simulink model "LinkageC"  (R2025b)
settings: Solver=VariableStepAuto  StartTime=0  StopTime=numPeriods*T  RelTol=1e-3  AbsTol=1e-3
values from neighbouring files (symbols this model uses):
  A_G = 56.801    [LinkageGeometrySetUp.m]    (also in LinkageGeometrySetUp_imp.m = 55; LinkageGeometry_Fabio_ver.m = 20)
  alpha_0 = deg2rad(0.5)    [Iteration.m]    (also in Iteration_geometry.m; StartUp.m)
  alpha_stall_static = deg2rad(13)    [Iteration.m]    (also in Iteration_geometry.m; StartUp.m)
  AR = b^2/A    [LinkageGeometry_Modify.m]    (also in StartUp.m)
  Cd_cf = 1.5    [Iteration.m]    (also in Iteration_geometry.m; StartUp.m)
  CordOut = linspace(CordOut_root, CordOut_tip, WingSecNum_Out)    [LinkageGeometry_Modify.m]    (also in StartUp.m)
  D = 0;" newline      "    return;" newline      "end" newline      "q = 0.5*rho*Vmag^2;" newline      "D = q*S*CD;" newline      "L = q*S*CL;" newline      "    [build_wing_template.m]
  del_t = t_tot/(numSample)    [InputSetUp.m]
  eta_s = 0.90    (= 0.9)    [Iteration.m]    (also in Iteration_geometry.m; StartUp.m)
  InboardCord = 0.35*L_D/0.037    [LinkageGeometry_Modify.m]    (also in StartUp.m = 0.4)
  k_inboard = k * InboardCord/meanCord    [LinkageGeometry_Modify.m]    (also in StartUp.m = 12.5663706144)
  k_outboard = k * CordOut/meanCord    [LinkageGeometry_Modify.m]    (also in StartUp.m)
  Ka = 10    [StartUp3_control.m]
  Km = 73    [StartUp3_control.m]
  L_C = (3.589/1.5)*L_D    [LinkageGeometrySetUp.m]    (also in LinkageGeometrySetUp_imp.m = (9.37/3.7)*L_D; LinkageGeometry_Fabio_ver.m = 0.07885)
  L_C1 = (2.445/1.5)*L_D    [LinkageGeometrySetUp.m]    (also in LinkageGeometrySetUp_imp.m = (5.91/3.7)*L_D; LinkageGeometry_Fabio_ver.m = 0.04893)
  L_D = L_D_val(iter)    [Iteration_geometry.m]    (also in LinkageGeometry_Fabio_ver.m = 0.03019; StartUp.m = 0.037)
  L_EF = (1.494/1.5)*L_D    [LinkageGeometrySetUp.m]    (also in LinkageGeometrySetUp_imp.m = (4.468/3.7)*L_D; LinkageGeometry_Fabio_ver.m = 0.036)
  L_EG = (1.265/1.5)*L_D    [LinkageGeometrySetUp.m]    (also in LinkageGeometrySetUp_imp.m = L_C2; LinkageGeometry_Fabio_ver.m = 0.03)
  L_F = (16.189/1.5)*L_D    [LinkageGeometrySetUp.m]    (also in LinkageGeometrySetUp_imp.m = (39.93/3.7)*L_D; LinkageGeometry_Fabio_ver.m = 0.364)
  L_FH = (1.002/1.5)*L_D    [LinkageGeometrySetUp.m]    (also in LinkageGeometrySetUp_imp.m = (2.842/3.7)*L_D; LinkageGeometry_Fabio_ver.m = 0.02)
  L_Fl = (16.118/1.5)*L_D    [LinkageGeometrySetUp.m]    (also in LinkageGeometrySetUp_imp.m = L_F; LinkageGeometry_Fabio_ver.m = 0.364)
  L_Fp = (4.051/1.5)*L_D    [LinkageGeometrySetUp.m]    (also in LinkageGeometrySetUp_imp.m = (9.99/3.7)*L_D; LinkageGeometry_Fabio_ver.m = 0.14288)
  L_GH = (1.129/1.5)*L_D    [LinkageGeometrySetUp.m]    (also in LinkageGeometrySetUp_imp.m = (3.046/3.7)*L_D; LinkageGeometry_Fabio_ver.m = 0.016)
  L_t = 0.5/100    (= 0.005)    [LinkageGeometrySetUp.m]    (also in LinkageGeometrySetUp_imp.m; LinkageGeometry_Fabio_ver.m; LinkageGeometry_Modify.m)
  L_tip = (19.334/1.5)*L_D    [LinkageGeometrySetUp.m]    (also in LinkageGeometrySetUp_imp.m = (43/3.7)*L_D; LinkageGeometry_Fabio_ver.m = 0.55)
  M_in_i = M_in/WingSecNum_In    (= 0.0341666666667)    [StartUp.m]
  M_ser = 0.02    [StartUp.m]
  mu = 1.81e-5    (= 1.81e-05)    [Iteration.m]    (also in Iteration_geometry.m; StartUp.m)
  noise_freq_cutoff = 20*ang_freq    [InputSetUp.m]
  P_ref = 10    [StartUp3_control.m]
  phase_data_lookup = phase_data_lookup(1:(end-1))    [StartUp.m]
  pitch_data_lookup = pitch_ts.Data(1:numSampPerT)    [InputSetUp.m]
  pitch_gain = linspace(0.1, 1, WingSecNum_Out)    [InputSetUp.m]
  pitch_lookup_input = 1    [Iteration.m]    (also in Iteration_geometry.m; StartUp.m)
  pitch_mean = deg2rad(20)    [Iteration.m]    (also in Iteration_geometry.m; Iteration_speed.m; StartUp.m = deg2rad(1); StartUp3_control.m = deg2rad(1))
  rho = 1.225    [StartUp.m]
  SectionWidth_In = L_Inboard/WingSecNum_In    [LinkageGeometry_Modify.m]    (also in StartUp.m = (L_Inboard/WingSecNum_In)*0.6)
  SectionWidth_Out = L_outboard/WingSecNum_Out    [LinkageGeometry_Modify.m]    (also in StartUp.m)
  SpeedControlYes = 1    [StartUp3_control.m]
  TorqueLimit = 7.2    [StartUp3_control.m]
  U = 0.1    [Iteration.m]    (also in Iteration_geometry.m; StartUp.m)
  xi = 0.0    (= 0)    [Iteration.m]    (also in Iteration_geometry.m; StartUp.m)
undefined symbols (not defined in the file or in its folder): angle_data_lookup, DiscIntNeverNeededParam, magnitude, Pivot, X, Y, Z
libraries: sm_lib x1370, nesl_utility x916, simulink x478, cstblocks x78, simulink_extras x10, slpidlib x2
(part 41 of 57)

== system LinkageC/Wing System (Festo)/Wing Tip/WingSeg_Out_6/1993dL&dT ==
  i : Inport
  inboard_yes? : Inport  Port=2
  AeroCalc : MATLAB Function  TreatAsAtomicUnit=on
  Discrete Derivative : simulink/Discrete/Discrete Derivative  gainval=1.0  ICPrevScaledInput=0.0  OutMin=[]  OutMax=[]  OutDataType=fixdt(1, 16)  OutScaling=2^-10  DoSatur=off
  Discrete Derivative1 : simulink/Discrete/Discrete Derivative  gainval=1.0  ICPrevScaledInput=0.0  OutMin=[]  OutMax=[]  OutDataType=fixdt(1, 16)  OutScaling=2^-10  DoSatur=off
  DocBlock : simulink/Model-Wide Utilities/DocBlock  DocumentType=Text
      content=|
      | Hello!
      |
      | Here's the idea behind this block:
      |
      | For force normal to plate (lift):
      | - dNc is applied at 1/4 cord location, normal to plate
      |     - it involves velocity at 3/4 cord
      | - dNa is applied at 2/4 cord location
      |     - involves speed at 2/4 cord (normal to plate component)
      | - dN = dNa + dNc
      |
      | For foce in chordwise direction (drag & thrust)
      | - dDcamber
      |     - drag due to camber
      | - dTs
      |     - thrust due to leading edge suction
      | - dDf
      |     - drag due to skin friciton
      | - dFx
      |     - net x direction force
      |
      |
      | --------------------special case (separated flow) ------------------------
      | When the attached flow range is exceeded, totally separated
      | flow is assumed to abruptly occur, for which condition all
      | chordwise forces are negligible (dFx = 0)
      | - dNc_sep = ...
      | - dNa_sep = 0.5*dNa
      |
      |
      | ----------------- summing result -----------------------------------------
      | - dL = dN*cos(theta) + dFx*sin(theta)
  External Force and Torque1 : sm_lib/Forces and Torques/External Force and Torque  EnableForceX=off  EnableForceY=on  EnableForceZ=on  EnableForce=off  ForceResolutionFrame=World  EnableTorqueX=off  EnableTorqueY=off  EnableTorqueZ=off  EnableTorque=off  TorqueResolutionFrame=AttachedFrame
  F1/4 : sm_lib/Frames and Transforms/Rigid Transform  RotationMethod=None  FollAlignAxisA=+X  BaseAlignAxisA=+Y  FollAlignAxisB=+Y  BaseAlignAxisB=+Z  RotationStandardAxis=+Z  RotationAngle=0  RotationAngleUnits=deg  RotationArbitraryAxis=[0 0 1]  RotationSequenceAxes=FollowerAxes  RotationSequence=XYX  RotationSequenceAngles=[0 0 0]  RotationSequenceAnglesUnits=deg  RotationMatrix=[1 0 0;0 1 0;0 0 1]  Quaternion=[1 0 0 0]  TranslationMethod=Cartesian  TranslationCartesianOffset=[-0.058333 0 0]  TranslationCartesianOffsetUnits=m  TranslationStandardAxis=+Z  TranslationStandardOffset=0  TranslationStandardOffsetUnits=m  TranslationROffset=0  TranslationROffsetUnits=m  TranslationThetaOffset=0  TranslationThetaOffsetUnits=deg  TranslationZOffset=0  TranslationZOffsetUnits=m
  F3/4 : sm_lib/Frames and Transforms/Rigid Transform  RotationMethod=None  FollAlignAxisA=+X  BaseAlignAxisA=+Y  FollAlignAxisB=+Y  BaseAlignAxisB=+Z  RotationStandardAxis=+Z  RotationAngle=0  RotationAngleUnits=deg  RotationArbitraryAxis=[0 0 1]  RotationSequenceAxes=FollowerAxes  RotationSequence=XYX  RotationSequenceAngles=[0 0 0]  RotationSequenceAnglesUnits=deg  RotationMatrix=[1 0 0;0 1 0;0 0 1]  Quaternion=[1 0 0 0]  TranslationMethod=Cartesian  TranslationCartesianOffset=[0.058333 0 0]  TranslationCartesianOffsetUnits=m  TranslationStandardAxis=+Z  TranslationStandardOffset=0  TranslationStandardOffsetUnits=m  TranslationROffset=0  TranslationROffsetUnits=m  TranslationThetaOffset=0  TranslationThetaOffsetUnits=deg  TranslationZOffset=0  TranslationZOffsetUnits=m
  LeadingEdge : sm_lib/Frames and Transforms/Rigid Transform  RotationMethod=None  FollAlignAxisA=+X  BaseAlignAxisA=+Y  FollAlignAxisB=+Y  BaseAlignAxisB=+Z  RotationStandardAxis=+Z  RotationAngle=0  RotationAngleUnits=deg  RotationArbitraryAxis=[0 0 1]  RotationSequenceAxes=FollowerAxes  RotationSequence=XYX  RotationSequenceAngles=[0 0 0]  RotationSequenceAnglesUnits=deg  RotationMatrix=[1 0 0;0 1 0;0 0 1]  Quaternion=[1 0 0 0]  TranslationMethod=Cartesian  TranslationCartesianOffset=[-0.11667 0 0]  TranslationCartesianOffsetUnits=m  TranslationStandardAxis=+Z  TranslationStandardOffset=0  TranslationStandardOffsetUnits=m  TranslationROffset=0  TranslationROffsetUnits=m  TranslationThetaOffset=0  TranslationThetaOffsetUnits=deg  TranslationZOffset=0  TranslationZOffsetUnits=m
  Memory : Memory
  PS-Simulink Converter1 : nesl_utility/PS-Simulink Converter  PhysicalDomain=network_engine_domain  SubClassName=ps_output  LeftPortType=input  RightPortType=output  PseudoPeriodic=off  Frequencies=[]  VectorFormat=inherit  Unit=inherit  AffineConversion=off
  PS-Simulink Converter3 : nesl_utility/PS-Simulink Converter  Commented=on  PhysicalDomain=network_engine_domain  SubClassName=ps_output  LeftPortType=input  RightPortType=output  PseudoPeriodic=off  Frequencies=[]  VectorFormat=inherit  Unit=inherit  AffineConversion=off
  PS-Simulink Converter4 : nesl_utility/PS-Simulink Converter  PhysicalDomain=network_engine_domain  SubClassName=ps_output  LeftPortType=input  RightPortType=output  PseudoPeriodic=off  Frequencies=[]  VectorFormat=inherit  Unit=inherit  AffineConversion=off
  PS-Simulink Converter5 : nesl_utility/PS-Simulink Converter  PhysicalDomain=network_engine_domain  SubClassName=ps_output  LeftPortType=input  RightPortType=output  PseudoPeriodic=off  Frequencies=[]  VectorFormat=inherit  Unit=inherit  AffineConversion=off
  PS-Simulink Converter6 : nesl_utility/PS-Simulink Converter  Commented=on  PhysicalDomain=network_engine_domain  SubClassName=ps_output  LeftPortType=input  RightPortType=output  PseudoPeriodic=off  Frequencies=[]  VectorFormat=inherit  Unit=inherit  AffineConversion=off
  Product : Product
  Product1 : Product
  Scope : Scope
  Simulink-PS Converter : nesl_utility/Simulink-PS Converter  PhysicalDomain=network_engine_domain  SubClassName=ps_input  LeftPortType=input  RightPortType=output  PseudoPeriodic=off  Frequencies=[]  NoiseDistribution=none  NoiseParameters=[]  Unit=1  AffineConversion=off  FilteringAndDerivatives=provide  SimscapeFilterOrder=1  InputFilterTimeConstant=0.001  UdotUserProvided=0
  Simulink-PS Converter1 : nesl_utility/Simulink-PS Converter  PhysicalDomain=network_engine_domain  SubClassName=ps_input  LeftPortType=input  RightPortType=output  PseudoPeriodic=off  Frequencies=[]  NoiseDistribution=none  NoiseParameters=[]  Unit=1  AffineConversion=off  FilteringAndDerivatives=provide  SimscapeFilterOrder=1  InputFilterTimeConstant=0.001  UdotUserProvided=0
  Simulink-PS Converter4 : nesl_utility/Simulink-PS Converter  Commented=on  PhysicalDomain=network_engine_domain  SubClassName=ps_input  LeftPortType=input  RightPortType=output  PseudoPeriodic=off  Frequencies=[]  NoiseDistribution=none  NoiseParameters=[]  Unit=1  AffineConversion=off  FilteringAndDerivatives=provide  SimscapeFilterOrder=1  InputFilterTimeConstant=0.001  UdotUserProvided=0
  Switch : Switch  Criteria=u2 > Threshold  SaturateOnIntegerOverflow=off  InputSameDT=off
  Transform Sensor : sm_lib/Frames and Transforms/Transform Sensor  MeasurementFrame=World  RotationSequence=XYX  SenseAngle=off  SenseAxis=off  SenseQ=off  SenseR=off  SenseRotationSequence=off  SenseOmegaX=off  SenseOmegaY=off  SenseOmegaZ=off  SenseOmega=off  SenseQDot=off  SenseRDot=off  SenseRotationSequenceDot=off  SenseAlphaX=off  SenseAlphaY=off  SenseAlphaZ=off  SenseAlpha=off  SenseQDDot=off  SenseRDDot=off  SenseX=off  SenseY=off  SenseZ=off  SenseXYZ=off  SenseRad=off  SenseAzim=off  SenseDist=off  SenseInc=off  SenseXDot=on  SenseYDot=on  SenseZDot=on  SenseXYZDot=off  SenseRadDot=off  SenseAzimDot=off  SenseDistDot=off  SenseIncDot=off  SenseXDDot=off  SenseYDDot=off  SenseZDDot=off  SenseXYZDDot=off  SenseRadDDot=off  SenseAzimDDot=off  SenseDistDDot=off  SenseIncDDot=off
  Transform Sensor1 : sm_lib/Frames and Transforms/Transform Sensor  MeasurementFrame=World  RotationSequence=XYX  SenseAngle=off  SenseAxis=off  SenseQ=off  SenseR=on  SenseRotationSequence=off  SenseOmegaX=off  SenseOmegaY=off  SenseOmegaZ=off  SenseOmega=off  SenseQDot=off  SenseRDot=off  SenseRotationSequenceDot=off  SenseAlphaX=off  SenseAlphaY=off  SenseAlphaZ=off  SenseAlpha=off  SenseQDDot=off  SenseRDDot=off  SenseX=off  SenseY=off  SenseZ=off  SenseXYZ=off  SenseRad=off  SenseAzim=off  SenseDist=off  SenseInc=off  SenseXDot=off  SenseYDot=on  SenseZDot=off  SenseXYZDot=off  SenseRadDot=off  SenseAzimDot=off  SenseDistDot=off  SenseIncDot=off  SenseXDDot=off  SenseYDDot=on  SenseZDDot=off  SenseXYZDDot=off  SenseRadDDot=off  SenseAzimDDot=off  SenseDistDDot=off  SenseIncDDot=off
  Transform Sensor2 : sm_lib/Frames and Transforms/Transform Sensor  MeasurementFrame=World  RotationSequence=XYX  SenseAngle=off  SenseAxis=off  SenseQ=off  SenseR=off  SenseRotationSequence=off  SenseOmegaX=off  SenseOmegaY=off  SenseOmegaZ=off  SenseOmega=off  SenseQDot=off  SenseRDot=off  SenseRotationSequenceDot=off  SenseAlphaX=off  SenseAlphaY=off  SenseAlphaZ=off  SenseAlpha=off  SenseQDDot=off  SenseRDDot=off  SenseX=off  SenseY=off  SenseZ=off  SenseXYZ=off  SenseRad=off  SenseAzim=off  SenseDist=off  SenseInc=off  SenseXDot=on  SenseYDot=on  SenseZDot=on  SenseXYZDot=off  SenseRadDot=off  SenseAzimDot=off  SenseDistDot=off  SenseIncDot=off  SenseXDDot=off  SenseYDDot=off  SenseZDDot=off  SenseXYZDDot=off  SenseRadDDot=off  SenseAzimDDot=off  SenseDistDDot=off  SenseIncDDot=off
  Transform Sensor3 : sm_lib/Frames and Transforms/Transform Sensor  MeasurementFrame=World  RotationSequence=XYX  SenseAngle=off  SenseAxis=off  SenseQ=off  SenseR=off  SenseRotationSequence=off  SenseOmegaX=off  SenseOmegaY=off  SenseOmegaZ=off  SenseOmega=off  SenseQDot=off  SenseRDot=off  SenseRotationSequenceDot=off  SenseAlphaX=off  SenseAlphaY=off  SenseAlphaZ=off  SenseAlpha=off  SenseQDDot=off  SenseRDDot=off  SenseX=off  SenseY=off  SenseZ=off  SenseXYZ=off  SenseRad=off  SenseAzim=off  SenseDist=off  SenseInc=off  SenseXDot=on  SenseYDot=on  SenseZDot=on  SenseXYZDot=off  SenseRadDot=off  SenseAzimDot=off  SenseDistDot=off  SenseIncDot=off  SenseXDDot=off  SenseYDDot=off  SenseZDDot=off  SenseXYZDDot=off  SenseRadDDot=off  SenseAzimDDot=off  SenseDistDDot=off  SenseIncDDot=off
  Varying Lowpass Filter : cstblocks/Linear Parameter Varying/Varying Lowpass Filter  N=2
  World Frame1 : sm_lib/Frames and Transforms/World Frame
  cutoff_freq(rad/s) : Constant  Value=noise_freq_cutoff
  h is positive when wing is low : Constant  Value=-1
  h is positive when wing is low1 : Constant  Value=-1
  pitch_lookup?(1=yes) : Constant  Value=pitch_lookup_input
  pitch_tip_in : FromWorkspace  VariableName=pitch_tip_in  SampleTime=del_t
  Cord2/4_F : PMIOPort  Side=Left
  dL : Outport
  dT : Outport  Port=2
  wires:
  [pitch_m] -> Switch/1
  pitch_tip_in/1 -> Switch/3  "pitch"
  pitch_lookup?(1=yes)/1 -> Switch/2
  cutoff_freq(rad/s)/1 -> Varying Lowpass Filter/2
  Memory/1 -> Varying Lowpass Filter/1
  Varying Lowpass Filter/1 -> AeroCalc/3(h_ddot)  "h_ddot_f"
  Product1/1 -> Memory/1  "h_ddot"
  PS-Simulink Converter1/1 -> Product1/1
  h is positive when wing is low1/1 -> Product1/2
  PS-Simulink Converter4/1 -> Product/1
  h is positive when wing is low/1 -> Product/2
  AeroCalc/3(stall_yes) -> Scope/1  "stall_if_positive"
  inboard_yes?/1 -> AeroCalc/5(in)
  Discrete Derivative1/1 -> AeroCalc/8(pitch_i_dd)
  Discrete Derivative/1 -> Discrete Derivative1/1, AeroCalc/7(pitch_i_d)
  i/1 -> AeroCalc/4(i)
  Switch/1 -> Discrete Derivative/1, AeroCalc/6(pitch_i)
  PS-Simulink Converter5/1 -> AeroCalc/1(R)  "R"
  Product/1 -> AeroCalc/2(h_dot)  "h_dot"
  AeroCalc/2(dT) -> Simulink-PS Converter1/1, dT/1  "dT"
  AeroCalc/1(dL) -> Simulink-PS Converter/1, dL/1  "dL"
  connections:
  Transform Sensor1/RConn4 -- PS-Simulink Converter1/LConn1
  Simulink-PS Converter1/RConn1 -- External Force and Torque1/LConn2
  F3/4/RConn1 -- Transform Sensor3/RConn1
  F1/4/RConn1 -- Transform Sensor/RConn1
  LeadingEdge/RConn1 -- Transform Sensor1/RConn1
  Transform Sensor1/RConn2 -- PS-Simulink Converter5/LConn1
  PS-Simulink Converter4/LConn1 -- Transform Sensor1/RConn3
  Transform Sensor2/RConn1 -- F3/4/LConn1 -- Cord2/4_F/RConn1 -- LeadingEdge/LConn1 -- F1/4/LConn1 -- External Force and Torque1/RConn1
  Simulink-PS Converter/RConn1 -- External Force and Torque1/LConn1
  Transform Sensor/LConn1 -- Transform Sensor2/LConn1 -- Transform Sensor3/LConn1 -- World Frame1/RConn1 -- Transform Sensor1/LConn1

== system LinkageC/Wing System (Festo)/Wing Tip/WingSeg_Out_7/1993dL&dT ==
  i : Inport
  inboard_yes? : Inport  Port=2
  AeroCalc : MATLAB Function  TreatAsAtomicUnit=on
  Discrete Derivative : simulink/Discrete/Discrete Derivative  gainval=1.0  ICPrevScaledInput=0.0  OutMin=[]  OutMax=[]  OutDataType=fixdt(1, 16)  OutScaling=2^-10  DoSatur=off
  Discrete Derivative1 : simulink/Discrete/Discrete Derivative  gainval=1.0  ICPrevScaledInput=0.0  OutMin=[]  OutMax=[]  OutDataType=fixdt(1, 16)  OutScaling=2^-10  DoSatur=off
  DocBlock : simulink/Model-Wide Utilities/DocBlock  DocumentType=Text
      content=|
      | Hello!
      |
      | Here's the idea behind this block:
      |
      | For force normal to plate (lift):
      | - dNc is applied at 1/4 cord location, normal to plate
      |     - it involves velocity at 3/4 cord
      | - dNa is applied at 2/4 cord location
      |     - involves speed at 2/4 cord (normal to plate component)
      | - dN = dNa + dNc
      |
      | For foce in chordwise direction (drag & thrust)
      | - dDcamber
      |     - drag due to camber
      | - dTs
      |     - thrust due to leading edge suction
      | - dDf
      |     - drag due to skin friciton
      | - dFx
      |     - net x direction force
      |
      |
      | --------------------special case (separated flow) ------------------------
      | When the attached flow range is exceeded, totally separated
      | flow is assumed to abruptly occur, for which condition all
      | chordwise forces are negligible (dFx = 0)
      | - dNc_sep = ...
      | - dNa_sep = 0.5*dNa
      |
      |
      | ----------------- summing result -----------------------------------------
      | - dL = dN*cos(theta) + dFx*sin(theta)
  External Force and Torque1 : sm_lib/Forces and Torques/External Force and Torque  EnableForceX=off  EnableForceY=on  EnableForceZ=on  EnableForce=off  ForceResolutionFrame=World  EnableTorqueX=off  EnableTorqueY=off  EnableTorqueZ=off  EnableTorque=off  TorqueResolutionFrame=AttachedFrame
  F1/4 : sm_lib/Frames and Transforms/Rigid Transform  RotationMethod=None  FollAlignAxisA=+X  BaseAlignAxisA=+Y  FollAlignAxisB=+Y  BaseAlignAxisB=+Z  RotationStandardAxis=+Z  RotationAngle=0  RotationAngleUnits=deg  RotationArbitraryAxis=[0 0 1]  RotationSequenceAxes=FollowerAxes  RotationSequence=XYX  RotationSequenceAngles=[0 0 0]  RotationSequenceAnglesUnits=deg  RotationMatrix=[1 0 0;0 1 0;0 0 1]  Quaternion=[1 0 0 0]  TranslationMethod=Cartesian  TranslationCartesianOffset=[-0.0525 0 0]  TranslationCartesianOffsetUnits=m  TranslationStandardAxis=+Z  TranslationStandardOffset=0  TranslationStandardOffsetUnits=m  TranslationROffset=0  TranslationROffsetUnits=m  TranslationThetaOffset=0  TranslationThetaOffsetUnits=deg  TranslationZOffset=0  TranslationZOffsetUnits=m
  F3/4 : sm_lib/Frames and Transforms/Rigid Transform  RotationMethod=None  FollAlignAxisA=+X  BaseAlignAxisA=+Y  FollAlignAxisB=+Y  BaseAlignAxisB=+Z  RotationStandardAxis=+Z  RotationAngle=0  RotationAngleUnits=deg  RotationArbitraryAxis=[0 0 1]  RotationSequenceAxes=FollowerAxes  RotationSequence=XYX  RotationSequenceAngles=[0 0 0]  RotationSequenceAnglesUnits=deg  RotationMatrix=[1 0 0;0 1 0;0 0 1]  Quaternion=[1 0 0 0]  TranslationMethod=Cartesian  TranslationCartesianOffset=[0.0525 0 0]  TranslationCartesianOffsetUnits=m  TranslationStandardAxis=+Z  TranslationStandardOffset=0  TranslationStandardOffsetUnits=m  TranslationROffset=0  TranslationROffsetUnits=m  TranslationThetaOffset=0  TranslationThetaOffsetUnits=deg  TranslationZOffset=0  TranslationZOffsetUnits=m
  LeadingEdge : sm_lib/Frames and Transforms/Rigid Transform  RotationMethod=None  FollAlignAxisA=+X  BaseAlignAxisA=+Y  FollAlignAxisB=+Y  BaseAlignAxisB=+Z  RotationStandardAxis=+Z  RotationAngle=0  RotationAngleUnits=deg  RotationArbitraryAxis=[0 0 1]  RotationSequenceAxes=FollowerAxes  RotationSequence=XYX  RotationSequenceAngles=[0 0 0]  RotationSequenceAnglesUnits=deg  RotationMatrix=[1 0 0;0 1 0;0 0 1]  Quaternion=[1 0 0 0]  TranslationMethod=Cartesian  TranslationCartesianOffset=[-0.105 0 0]  TranslationCartesianOffsetUnits=m  TranslationStandardAxis=+Z  TranslationStandardOffset=0  TranslationStandardOffsetUnits=m  TranslationROffset=0  TranslationROffsetUnits=m  TranslationThetaOffset=0  TranslationThetaOffsetUnits=deg  TranslationZOffset=0  TranslationZOffsetUnits=m
  Memory : Memory
  PS-Simulink Converter1 : nesl_utility/PS-Simulink Converter  PhysicalDomain=network_engine_domain  SubClassName=ps_output  LeftPortType=input  RightPortType=output  PseudoPeriodic=off  Frequencies=[]  VectorFormat=inherit  Unit=inherit  AffineConversion=off
  PS-Simulink Converter3 : nesl_utility/PS-Simulink Converter  Commented=on  PhysicalDomain=network_engine_domain  SubClassName=ps_output  LeftPortType=input  RightPortType=output  PseudoPeriodic=off  Frequencies=[]  VectorFormat=inherit  Unit=inherit  AffineConversion=off
  PS-Simulink Converter4 : nesl_utility/PS-Simulink Converter  PhysicalDomain=network_engine_domain  SubClassName=ps_output  LeftPortType=input  RightPortType=output  PseudoPeriodic=off  Frequencies=[]  VectorFormat=inherit  Unit=inherit  AffineConversion=off
  PS-Simulink Converter5 : nesl_utility/PS-Simulink Converter  PhysicalDomain=network_engine_domain  SubClassName=ps_output  LeftPortType=input  RightPortType=output  PseudoPeriodic=off  Frequencies=[]  VectorFormat=inherit  Unit=inherit  AffineConversion=off
  PS-Simulink Converter6 : nesl_utility/PS-Simulink Converter  Commented=on  PhysicalDomain=network_engine_domain  SubClassName=ps_output  LeftPortType=input  RightPortType=output  PseudoPeriodic=off  Frequencies=[]  VectorFormat=inherit  Unit=inherit  AffineConversion=off
  Product : Product
  Product1 : Product
  Scope : Scope
  Simulink-PS Converter : nesl_utility/Simulink-PS Converter  PhysicalDomain=network_engine_domain  SubClassName=ps_input  LeftPortType=input  RightPortType=output  PseudoPeriodic=off  Frequencies=[]  NoiseDistribution=none  NoiseParameters=[]  Unit=1  AffineConversion=off  FilteringAndDerivatives=provide  SimscapeFilterOrder=1  InputFilterTimeConstant=0.001  UdotUserProvided=0
  Simulink-PS Converter1 : nesl_utility/Simulink-PS Converter  PhysicalDomain=network_engine_domain  SubClassName=ps_input  LeftPortType=input  RightPortType=output  PseudoPeriodic=off  Frequencies=[]  NoiseDistribution=none  NoiseParameters=[]  Unit=1  AffineConversion=off  FilteringAndDerivatives=provide  SimscapeFilterOrder=1  InputFilterTimeConstant=0.001  UdotUserProvided=0
  Simulink-PS Converter4 : nesl_utility/Simulink-PS Converter  Commented=on  PhysicalDomain=network_engine_domain  SubClassName=ps_input  LeftPortType=input  RightPortType=output  PseudoPeriodic=off  Frequencies=[]  NoiseDistribution=none  NoiseParameters=[]  Unit=1  AffineConversion=off  FilteringAndDerivatives=provide  SimscapeFilterOrder=1  InputFilterTimeConstant=0.001  UdotUserProvided=0
  Switch : Switch  Criteria=u2 > Threshold  SaturateOnIntegerOverflow=off  InputSameDT=off
  Transform Sensor : sm_lib/Frames and Transforms/Transform Sensor  MeasurementFrame=World  RotationSequence=XYX  SenseAngle=off  SenseAxis=off  SenseQ=off  SenseR=off  SenseRotationSequence=off  SenseOmegaX=off  SenseOmegaY=off  SenseOmegaZ=off  SenseOmega=off  SenseQDot=off  SenseRDot=off  SenseRotationSequenceDot=off  SenseAlphaX=off  SenseAlphaY=off  SenseAlphaZ=off  SenseAlpha=off  SenseQDDot=off  SenseRDDot=off  SenseX=off  SenseY=off  SenseZ=off  SenseXYZ=off  SenseRad=off  SenseAzim=off  SenseDist=off  SenseInc=off  SenseXDot=on  SenseYDot=on  SenseZDot=on  SenseXYZDot=off  SenseRadDot=off  SenseAzimDot=off  SenseDistDot=off  SenseIncDot=off  SenseXDDot=off  SenseYDDot=off  SenseZDDot=off  SenseXYZDDot=off  SenseRadDDot=off  SenseAzimDDot=off  SenseDistDDot=off  SenseIncDDot=off
  Transform Sensor1 : sm_lib/Frames and Transforms/Transform Sensor  MeasurementFrame=World  RotationSequence=XYX  SenseAngle=off  SenseAxis=off  SenseQ=off  SenseR=on  SenseRotationSequence=off  SenseOmegaX=off  SenseOmegaY=off  SenseOmegaZ=off  SenseOmega=off  SenseQDot=off  SenseRDot=off  SenseRotationSequenceDot=off  SenseAlphaX=off  SenseAlphaY=off  SenseAlphaZ=off  SenseAlpha=off  SenseQDDot=off  SenseRDDot=off  SenseX=off  SenseY=off  SenseZ=off  SenseXYZ=off  SenseRad=off  SenseAzim=off  SenseDist=off  SenseInc=off  SenseXDot=off  SenseYDot=on  SenseZDot=off  SenseXYZDot=off  SenseRadDot=off  SenseAzimDot=off  SenseDistDot=off  SenseIncDot=off  SenseXDDot=off  SenseYDDot=on  SenseZDDot=off  SenseXYZDDot=off  SenseRadDDot=off  SenseAzimDDot=off  SenseDistDDot=off  SenseIncDDot=off
  Transform Sensor2 : sm_lib/Frames and Transforms/Transform Sensor  MeasurementFrame=World  RotationSequence=XYX  SenseAngle=off  SenseAxis=off  SenseQ=off  SenseR=off  SenseRotationSequence=off  SenseOmegaX=off  SenseOmegaY=off  SenseOmegaZ=off  SenseOmega=off  SenseQDot=off  SenseRDot=off  SenseRotationSequenceDot=off  SenseAlphaX=off  SenseAlphaY=off  SenseAlphaZ=off  SenseAlpha=off  SenseQDDot=off  SenseRDDot=off  SenseX=off  SenseY=off  SenseZ=off  SenseXYZ=off  SenseRad=off  SenseAzim=off  SenseDist=off  SenseInc=off  SenseXDot=on  SenseYDot=on  SenseZDot=on  SenseXYZDot=off  SenseRadDot=off  SenseAzimDot=off  SenseDistDot=off  SenseIncDot=off  SenseXDDot=off  SenseYDDot=off  SenseZDDot=off  SenseXYZDDot=off  SenseRadDDot=off  SenseAzimDDot=off  SenseDistDDot=off  SenseIncDDot=off
  Transform Sensor3 : sm_lib/Frames and Transforms/Transform Sensor  MeasurementFrame=World  RotationSequence=XYX  SenseAngle=off  SenseAxis=off  SenseQ=off  SenseR=off  SenseRotationSequence=off  SenseOmegaX=off  SenseOmegaY=off  SenseOmegaZ=off  SenseOmega=off  SenseQDot=off  SenseRDot=off  SenseRotationSequenceDot=off  SenseAlphaX=off  SenseAlphaY=off  SenseAlphaZ=off  SenseAlpha=off  SenseQDDot=off  SenseRDDot=off  SenseX=off  SenseY=off  SenseZ=off  SenseXYZ=off  SenseRad=off  SenseAzim=off  SenseDist=off  SenseInc=off  SenseXDot=on  SenseYDot=on  SenseZDot=on  SenseXYZDot=off  SenseRadDot=off  SenseAzimDot=off  SenseDistDot=off  SenseIncDot=off  SenseXDDot=off  SenseYDDot=off  SenseZDDot=off  SenseXYZDDot=off  SenseRadDDot=off  SenseAzimDDot=off  SenseDistDDot=off  SenseIncDDot=off
  Varying Lowpass Filter : cstblocks/Linear Parameter Varying/Varying Lowpass Filter  N=2
  World Frame1 : sm_lib/Frames and Transforms/World Frame
  cutoff_freq(rad/s) : Constant  Value=noise_freq_cutoff
  h is positive when wing is low : Constant  Value=-1
  h is positive when wing is low1 : Constant  Value=-1
  pitch_lookup?(1=yes) : Constant  Value=pitch_lookup_input
  pitch_tip_in : FromWorkspace  VariableName=pitch_tip_in  SampleTime=del_t
  Cord2/4_F : PMIOPort  Side=Left
  dL : Outport
  dT : Outport  Port=2
  wires:
  [pitch_m] -> Switch/1
  pitch_tip_in/1 -> Switch/3  "pitch"
  pitch_lookup?(1=yes)/1 -> Switch/2
  cutoff_freq(rad/s)/1 -> Varying Lowpass Filter/2
  Memory/1 -> Varying Lowpass Filter/1
  Varying Lowpass Filter/1 -> AeroCalc/3(h_ddot)  "h_ddot_f"
  Product1/1 -> Memory/1  "h_ddot"
  PS-Simulink Converter1/1 -> Product1/1
  h is positive when wing is low1/1 -> Product1/2
  PS-Simulink Converter4/1 -> Product/1
  h is positive when wing is low/1 -> Product/2
  AeroCalc/3(stall_yes) -> Scope/1  "stall_if_positive"
  inboard_yes?/1 -> AeroCalc/5(in)
  Discrete Derivative1/1 -> AeroCalc/8(pitch_i_dd)
  Discrete Derivative/1 -> Discrete Derivative1/1, AeroCalc/7(pitch_i_d)
  i/1 -> AeroCalc/4(i)
  Switch/1 -> Discrete Derivative/1, AeroCalc/6(pitch_i)
  PS-Simulink Converter5/1 -> AeroCalc/1(R)  "R"
  Product/1 -> AeroCalc/2(h_dot)  "h_dot"
  AeroCalc/2(dT) -> Simulink-PS Converter1/1, dT/1  "dT"
  AeroCalc/1(dL) -> Simulink-PS Converter/1, dL/1  "dL"
  connections:
  Transform Sensor1/RConn4 -- PS-Simulink Converter1/LConn1
  Simulink-PS Converter1/RConn1 -- External Force and Torque1/LConn2
  F3/4/RConn1 -- Transform Sensor3/RConn1
  F1/4/RConn1 -- Transform Sensor/RConn1
  LeadingEdge/RConn1 -- Transform Sensor1/RConn1
  Transform Sensor1/RConn2 -- PS-Simulink Converter5/LConn1
  PS-Simulink Converter4/LConn1 -- Transform Sensor1/RConn3
  Transform Sensor2/RConn1 -- F3/4/LConn1 -- Cord2/4_F/RConn1 -- LeadingEdge/LConn1 -- F1/4/LConn1 -- External Force and Torque1/RConn1
  Simulink-PS Converter/RConn1 -- External Force and Torque1/LConn1
  Transform Sensor/LConn1 -- Transform Sensor2/LConn1 -- Transform Sensor3/LConn1 -- World Frame1/RConn1 -- Transform Sensor1/LConn1

== system LinkageC/Wing System (Festo)/Wing Tip/WingSeg_Out_8/1993dL&dT ==
  i : Inport
  inboard_yes? : Inport  Port=2
  AeroCalc : MATLAB Function  TreatAsAtomicUnit=on
  Discrete Derivative : simulink/Discrete/Discrete Derivative  gainval=1.0  ICPrevScaledInput=0.0  OutMin=[]  OutMax=[]  OutDataType=fixdt(1, 16)  OutScaling=2^-10  DoSatur=off
  Discrete Derivative1 : simulink/Discrete/Discrete Derivative  gainval=1.0  ICPrevScaledInput=0.0  OutMin=[]  OutMax=[]  OutDataType=fixdt(1, 16)  OutScaling=2^-10  DoSatur=off
  DocBlock : simulink/Model-Wide Utilities/DocBlock  DocumentType=Text
      content=|
      | Hello!
      |
      | Here's the idea behind this block:
      |
      | For force normal to plate (lift):
      | - dNc is applied at 1/4 cord location, normal to plate
      |     - it involves velocity at 3/4 cord
      | - dNa is applied at 2/4 cord location
      |     - involves speed at 2/4 cord (normal to plate component)
      | - dN = dNa + dNc
      |
      | For foce in chordwise direction (drag & thrust)
      | - dDcamber
      |     - drag due to camber
      | - dTs
      |     - thrust due to leading edge suction
      | - dDf
      |     - drag due to skin friciton
      | - dFx
      |     - net x direction force
      |
      |
      | --------------------special case (separated flow) ------------------------
      | When the attached flow range is exceeded, totally separated
      | flow is assumed to abruptly occur, for which condition all
      | chordwise forces are negligible (dFx = 0)
      | - dNc_sep = ...
      | - dNa_sep = 0.5*dNa
      |
      |
      | ----------------- summing result -----------------------------------------
      | - dL = dN*cos(theta) + dFx*sin(theta)
  External Force and Torque1 : sm_lib/Forces and Torques/External Force and Torque  EnableForceX=off  EnableForceY=on  EnableForceZ=on  EnableForce=off  ForceResolutionFrame=World  EnableTorqueX=off  EnableTorqueY=off  EnableTorqueZ=off  EnableTorque=off  TorqueResolutionFrame=AttachedFrame
  F1/4 : sm_lib/Frames and Transforms/Rigid Transform  RotationMethod=None  FollAlignAxisA=+X  BaseAlignAxisA=+Y  FollAlignAxisB=+Y  BaseAlignAxisB=+Z  RotationStandardAxis=+Z  RotationAngle=0  RotationAngleUnits=deg  RotationArbitraryAxis=[0 0 1]  RotationSequenceAxes=FollowerAxes  RotationSequence=XYX  RotationSequenceAngles=[0 0 0]  RotationSequenceAnglesUnits=deg  RotationMatrix=[1 0 0;0 1 0;0 0 1]  Quaternion=[1 0 0 0]  TranslationMethod=Cartesian  TranslationCartesianOffset=[-0.046667 0 0]  TranslationCartesianOffsetUnits=m  TranslationStandardAxis=+Z  TranslationStandardOffset=0  TranslationStandardOffsetUnits=m  TranslationROffset=0  TranslationROffsetUnits=m  TranslationThetaOffset=0  TranslationThetaOffsetUnits=deg  TranslationZOffset=0  TranslationZOffsetUnits=m
  F3/4 : sm_lib/Frames and Transforms/Rigid Transform  RotationMethod=None  FollAlignAxisA=+X  BaseAlignAxisA=+Y  FollAlignAxisB=+Y  BaseAlignAxisB=+Z  RotationStandardAxis=+Z  RotationAngle=0  RotationAngleUnits=deg  RotationArbitraryAxis=[0 0 1]  RotationSequenceAxes=FollowerAxes  RotationSequence=XYX  RotationSequenceAngles=[0 0 0]  RotationSequenceAnglesUnits=deg  RotationMatrix=[1 0 0;0 1 0;0 0 1]  Quaternion=[1 0 0 0]  TranslationMethod=Cartesian  TranslationCartesianOffset=[0.046667 0 0]  TranslationCartesianOffsetUnits=m  TranslationStandardAxis=+Z  TranslationStandardOffset=0  TranslationStandardOffsetUnits=m  TranslationROffset=0  TranslationROffsetUnits=m  TranslationThetaOffset=0  TranslationThetaOffsetUnits=deg  TranslationZOffset=0  TranslationZOffsetUnits=m
  LeadingEdge : sm_lib/Frames and Transforms/Rigid Transform  RotationMethod=None  FollAlignAxisA=+X  BaseAlignAxisA=+Y  FollAlignAxisB=+Y  BaseAlignAxisB=+Z  RotationStandardAxis=+Z  RotationAngle=0  RotationAngleUnits=deg  RotationArbitraryAxis=[0 0 1]  RotationSequenceAxes=FollowerAxes  RotationSequence=XYX  RotationSequenceAngles=[0 0 0]  RotationSequenceAnglesUnits=deg  RotationMatrix=[1 0 0;0 1 0;0 0 1]  Quaternion=[1 0 0 0]  TranslationMethod=Cartesian  TranslationCartesianOffset=[-0.093333 0 0]  TranslationCartesianOffsetUnits=m  TranslationStandardAxis=+Z  TranslationStandardOffset=0  TranslationStandardOffsetUnits=m  TranslationROffset=0  TranslationROffsetUnits=m  TranslationThetaOffset=0  TranslationThetaOffsetUnits=deg  TranslationZOffset=0  TranslationZOffsetUnits=m
  Memory : Memory
  PS-Simulink Converter1 : nesl_utility/PS-Simulink Converter  PhysicalDomain=network_engine_domain  SubClassName=ps_output  LeftPortType=input  RightPortType=output  PseudoPeriodic=off  Frequencies=[]  VectorFormat=inherit  Unit=inherit  AffineConversion=off
  PS-Simulink Converter3 : nesl_utility/PS-Simulink Converter  Commented=on  PhysicalDomain=network_engine_domain  SubClassName=ps_output  LeftPortType=input  RightPortType=output  PseudoPeriodic=off  Frequencies=[]  VectorFormat=inherit  Unit=inherit  AffineConversion=off
  PS-Simulink Converter4 : nesl_utility/PS-Simulink Converter  PhysicalDomain=network_engine_domain  SubClassName=ps_output  LeftPortType=input  RightPortType=output  PseudoPeriodic=off  Frequencies=[]  VectorFormat=inherit  Unit=inherit  AffineConversion=off
  PS-Simulink Converter5 : nesl_utility/PS-Simulink Converter  PhysicalDomain=network_engine_domain  SubClassName=ps_output  LeftPortType=input  RightPortType=output  PseudoPeriodic=off  Frequencies=[]  VectorFormat=inherit  Unit=inherit  AffineConversion=off
  PS-Simulink Converter6 : nesl_utility/PS-Simulink Converter  Commented=on  PhysicalDomain=network_engine_domain  SubClassName=ps_output  LeftPortType=input  RightPortType=output  PseudoPeriodic=off  Frequencies=[]  VectorFormat=inherit  Unit=inherit  AffineConversion=off
  Product : Product
  Product1 : Product
  Scope : Scope
  Simulink-PS Converter : nesl_utility/Simulink-PS Converter  PhysicalDomain=network_engine_domain  SubClassName=ps_input  LeftPortType=input  RightPortType=output  PseudoPeriodic=off  Frequencies=[]  NoiseDistribution=none  NoiseParameters=[]  Unit=1  AffineConversion=off  FilteringAndDerivatives=provide  SimscapeFilterOrder=1  InputFilterTimeConstant=0.001  UdotUserProvided=0
  Simulink-PS Converter1 : nesl_utility/Simulink-PS Converter  PhysicalDomain=network_engine_domain  SubClassName=ps_input  LeftPortType=input  RightPortType=output  PseudoPeriodic=off  Frequencies=[]  NoiseDistribution=none  NoiseParameters=[]  Unit=1  AffineConversion=off  FilteringAndDerivatives=provide  SimscapeFilterOrder=1  InputFilterTimeConstant=0.001  UdotUserProvided=0
  Simulink-PS Converter4 : nesl_utility/Simulink-PS Converter  Commented=on  PhysicalDomain=network_engine_domain  SubClassName=ps_input  LeftPortType=input  RightPortType=output  PseudoPeriodic=off  Frequencies=[]  NoiseDistribution=none  NoiseParameters=[]  Unit=1  AffineConversion=off  FilteringAndDerivatives=provide  SimscapeFilterOrder=1  InputFilterTimeConstant=0.001  UdotUserProvided=0
  Switch : Switch  Criteria=u2 > Threshold  SaturateOnIntegerOverflow=off  InputSameDT=off
  Transform Sensor : sm_lib/Frames and Transforms/Transform Sensor  MeasurementFrame=World  RotationSequence=XYX  SenseAngle=off  SenseAxis=off  SenseQ=off  SenseR=off  SenseRotationSequence=off  SenseOmegaX=off  SenseOmegaY=off  SenseOmegaZ=off  SenseOmega=off  SenseQDot=off  SenseRDot=off  SenseRotationSequenceDot=off  SenseAlphaX=off  SenseAlphaY=off  SenseAlphaZ=off  SenseAlpha=off  SenseQDDot=off  SenseRDDot=off  SenseX=off  SenseY=off  SenseZ=off  SenseXYZ=off  SenseRad=off  SenseAzim=off  SenseDist=off  SenseInc=off  SenseXDot=on  SenseYDot=on  SenseZDot=on  SenseXYZDot=off  SenseRadDot=off  SenseAzimDot=off  SenseDistDot=off  SenseIncDot=off  SenseXDDot=off  SenseYDDot=off  SenseZDDot=off  SenseXYZDDot=off  SenseRadDDot=off  SenseAzimDDot=off  SenseDistDDot=off  SenseIncDDot=off
  Transform Sensor1 : sm_lib/Frames and Transforms/Transform Sensor  MeasurementFrame=World  RotationSequence=XYX  SenseAngle=off  SenseAxis=off  SenseQ=off  SenseR=on  SenseRotationSequence=off  SenseOmegaX=off  SenseOmegaY=off  SenseOmegaZ=off  SenseOmega=off  SenseQDot=off  SenseRDot=off  SenseRotationSequenceDot=off  SenseAlphaX=off  SenseAlphaY=off  SenseAlphaZ=off  SenseAlpha=off  SenseQDDot=off  SenseRDDot=off  SenseX=off  SenseY=off  SenseZ=off  SenseXYZ=off  SenseRad=off  SenseAzim=off  SenseDist=off  SenseInc=off  SenseXDot=off  SenseYDot=on  SenseZDot=off  SenseXYZDot=off  SenseRadDot=off  SenseAzimDot=off  SenseDistDot=off  SenseIncDot=off  SenseXDDot=off  SenseYDDot=on  SenseZDDot=off  SenseXYZDDot=off  SenseRadDDot=off  SenseAzimDDot=off  SenseDistDDot=off  SenseIncDDot=off
  Transform Sensor2 : sm_lib/Frames and Transforms/Transform Sensor  MeasurementFrame=World  RotationSequence=XYX  SenseAngle=off  SenseAxis=off  SenseQ=off  SenseR=off  SenseRotationSequence=off  SenseOmegaX=off  SenseOmegaY=off  SenseOmegaZ=off  SenseOmega=off  SenseQDot=off  SenseRDot=off  SenseRotationSequenceDot=off  SenseAlphaX=off  SenseAlphaY=off  SenseAlphaZ=off  SenseAlpha=off  SenseQDDot=off  SenseRDDot=off  SenseX=off  SenseY=off  SenseZ=off  SenseXYZ=off  SenseRad=off  SenseAzim=off  SenseDist=off  SenseInc=off  SenseXDot=on  SenseYDot=on  SenseZDot=on  SenseXYZDot=off  SenseRadDot=off  SenseAzimDot=off  SenseDistDot=off  SenseIncDot=off  SenseXDDot=off  SenseYDDot=off  SenseZDDot=off  SenseXYZDDot=off  SenseRadDDot=off  SenseAzimDDot=off  SenseDistDDot=off  SenseIncDDot=off
  Transform Sensor3 : sm_lib/Frames and Transforms/Transform Sensor  MeasurementFrame=World  RotationSequence=XYX  SenseAngle=off  SenseAxis=off  SenseQ=off  SenseR=off  SenseRotationSequence=off  SenseOmegaX=off  SenseOmegaY=off  SenseOmegaZ=off  SenseOmega=off  SenseQDot=off  SenseRDot=off  SenseRotationSequenceDot=off  SenseAlphaX=off  SenseAlphaY=off  SenseAlphaZ=off  SenseAlpha=off  SenseQDDot=off  SenseRDDot=off  SenseX=off  SenseY=off  SenseZ=off  SenseXYZ=off  SenseRad=off  SenseAzim=off  SenseDist=off  SenseInc=off  SenseXDot=on  SenseYDot=on  SenseZDot=on  SenseXYZDot=off  SenseRadDot=off  SenseAzimDot=off  SenseDistDot=off  SenseIncDot=off  SenseXDDot=off  SenseYDDot=off  SenseZDDot=off  SenseXYZDDot=off  SenseRadDDot=off  SenseAzimDDot=off  SenseDistDDot=off  SenseIncDDot=off
  Varying Lowpass Filter : cstblocks/Linear Parameter Varying/Varying Lowpass Filter  N=2
  World Frame1 : sm_lib/Frames and Transforms/World Frame
  cutoff_freq(rad/s) : Constant  Value=noise_freq_cutoff
  h is positive when wing is low : Constant  Value=-1
  h is positive when wing is low1 : Constant  Value=-1
  pitch_lookup?(1=yes) : Constant  Value=pitch_lookup_input
  pitch_tip_in : FromWorkspace  VariableName=pitch_tip_in  SampleTime=del_t
  Cord2/4_F : PMIOPort  Side=Left
  dL : Outport
  dT : Outport  Port=2
  wires:
  [pitch_m] -> Switch/1
  pitch_tip_in/1 -> Switch/3  "pitch"
  pitch_lookup?(1=yes)/1 -> Switch/2
  cutoff_freq(rad/s)/1 -> Varying Lowpass Filter/2
  Memory/1 -> Varying Lowpass Filter/1
  Varying Lowpass Filter/1 -> AeroCalc/3(h_ddot)  "h_ddot_f"
  Product1/1 -> Memory/1  "h_ddot"
  PS-Simulink Converter1/1 -> Product1/1
  h is positive when wing is low1/1 -> Product1/2
  PS-Simulink Converter4/1 -> Product/1
  h is positive when wing is low/1 -> Product/2
  AeroCalc/3(stall_yes) -> Scope/1  "stall_if_positive"
  inboard_yes?/1 -> AeroCalc/5(in)
  Discrete Derivative1/1 -> AeroCalc/8(pitch_i_dd)
  Discrete Derivative/1 -> Discrete Derivative1/1, AeroCalc/7(pitch_i_d)
  i/1 -> AeroCalc/4(i)
  Switch/1 -> Discrete Derivative/1, AeroCalc/6(pitch_i)
  PS-Simulink Converter5/1 -> AeroCalc/1(R)  "R"
  Product/1 -> AeroCalc/2(h_dot)  "h_dot"
  AeroCalc/2(dT) -> Simulink-PS Converter1/1, dT/1  "dT"
  AeroCalc/1(dL) -> Simulink-PS Converter/1, dL/1  "dL"
  connections:
  Transform Sensor1/RConn4 -- PS-Simulink Converter1/LConn1
  Simulink-PS Converter1/RConn1 -- External Force and Torque1/LConn2
  F3/4/RConn1 -- Transform Sensor3/RConn1
  F1/4/RConn1 -- Transform Sensor/RConn1
  LeadingEdge/RConn1 -- Transform Sensor1/RConn1
  Transform Sensor1/RConn2 -- PS-Simulink Converter5/LConn1
  PS-Simulink Converter4/LConn1 -- Transform Sensor1/RConn3
  Transform Sensor2/RConn1 -- F3/4/LConn1 -- Cord2/4_F/RConn1 -- LeadingEdge/LConn1 -- F1/4/LConn1 -- External Force and Torque1/RConn1
  Simulink-PS Converter/RConn1 -- External Force and Torque1/LConn1
  Transform Sensor/LConn1 -- Transform Sensor2/LConn1 -- Transform Sensor3/LConn1 -- World Frame1/RConn1 -- Transform Sensor1/LConn1

== system LinkageC/Wing System (Festo)/Wing Tip/WingSeg_Out_9/1993dL&dT ==
  i : Inport
  inboard_yes? : Inport  Port=2
  AeroCalc : MATLAB Function  TreatAsAtomicUnit=on
  Discrete Derivative : simulink/Discrete/Discrete Derivative  gainval=1.0  ICPrevScaledInput=0.0  OutMin=[]  OutMax=[]  OutDataType=fixdt(1, 16)  OutScaling=2^-10  DoSatur=off
  Discrete Derivative1 : simulink/Discrete/Discrete Derivative  gainval=1.0  ICPrevScaledInput=0.0  OutMin=[]  OutMax=[]  OutDataType=fixdt(1, 16)  OutScaling=2^-10  DoSatur=off
  DocBlock : simulink/Model-Wide Utilities/DocBlock  DocumentType=Text
      content=|
      | Hello!
      |
      | Here's the idea behind this block:
      |
      | For force normal to plate (lift):
      | - dNc is applied at 1/4 cord location, normal to plate
      |     - it involves velocity at 3/4 cord
      | - dNa is applied at 2/4 cord location
      |     - involves speed at 2/4 cord (normal to plate component)
      | - dN = dNa + dNc
      |
      | For foce in chordwise direction (drag & thrust)
      | - dDcamber
      |     - drag due to camber
      | - dTs
      |     - thrust due to leading edge suction
      | - dDf
      |     - drag due to skin friciton
      | - dFx
      |     - net x direction force
      |
      |
      | --------------------special case (separated flow) ------------------------
      | When the attached flow range is exceeded, totally separated
      | flow is assumed to abruptly occur, for which condition all
      | chordwise forces are negligible (dFx = 0)
      | - dNc_sep = ...
      | - dNa_sep = 0.5*dNa
      |
      |
      | ----------------- summing result -----------------------------------------
      | - dL = dN*cos(theta) + dFx*sin(theta)
  External Force and Torque1 : sm_lib/Forces and Torques/External Force and Torque  EnableForceX=off  EnableForceY=on  EnableForceZ=on  EnableForce=off  ForceResolutionFrame=World  EnableTorqueX=off  EnableTorqueY=off  EnableTorqueZ=off  EnableTorque=off  TorqueResolutionFrame=AttachedFrame
  F1/4 : sm_lib/Frames and Transforms/Rigid Transform  RotationMethod=None  FollAlignAxisA=+X  BaseAlignAxisA=+Y  FollAlignAxisB=+Y  BaseAlignAxisB=+Z  RotationStandardAxis=+Z  RotationAngle=0  RotationAngleUnits=deg  RotationArbitraryAxis=[0 0 1]  RotationSequenceAxes=FollowerAxes  RotationSequence=XYX  RotationSequenceAngles=[0 0 0]  RotationSequenceAnglesUnits=deg  RotationMatrix=[1 0 0;0 1 0;0 0 1]  Quaternion=[1 0 0 0]  TranslationMethod=Cartesian  TranslationCartesianOffset=[-0.040833 0 0]  TranslationCartesianOffsetUnits=m  TranslationStandardAxis=+Z  TranslationStandardOffset=0  TranslationStandardOffsetUnits=m  TranslationROffset=0  TranslationROffsetUnits=m  TranslationThetaOffset=0  TranslationThetaOffsetUnits=deg  TranslationZOffset=0  TranslationZOffsetUnits=m
  F3/4 : sm_lib/Frames and Transforms/Rigid Transform  RotationMethod=None  FollAlignAxisA=+X  BaseAlignAxisA=+Y  FollAlignAxisB=+Y  BaseAlignAxisB=+Z  RotationStandardAxis=+Z  RotationAngle=0  RotationAngleUnits=deg  RotationArbitraryAxis=[0 0 1]  RotationSequenceAxes=FollowerAxes  RotationSequence=XYX  RotationSequenceAngles=[0 0 0]  RotationSequenceAnglesUnits=deg  RotationMatrix=[1 0 0;0 1 0;0 0 1]  Quaternion=[1 0 0 0]  TranslationMethod=Cartesian  TranslationCartesianOffset=[0.040833 0 0]  TranslationCartesianOffsetUnits=m  TranslationStandardAxis=+Z  TranslationStandardOffset=0  TranslationStandardOffsetUnits=m  TranslationROffset=0  TranslationROffsetUnits=m  TranslationThetaOffset=0  TranslationThetaOffsetUnits=deg  TranslationZOffset=0  TranslationZOffsetUnits=m
  LeadingEdge : sm_lib/Frames and Transforms/Rigid Transform  RotationMethod=None  FollAlignAxisA=+X  BaseAlignAxisA=+Y  FollAlignAxisB=+Y  BaseAlignAxisB=+Z  RotationStandardAxis=+Z  RotationAngle=0  RotationAngleUnits=deg  RotationArbitraryAxis=[0 0 1]  RotationSequenceAxes=FollowerAxes  RotationSequence=XYX  RotationSequenceAngles=[0 0 0]  RotationSequenceAnglesUnits=deg  RotationMatrix=[1 0 0;0 1 0;0 0 1]  Quaternion=[1 0 0 0]  TranslationMethod=Cartesian  TranslationCartesianOffset=[-0.081667 0 0]  TranslationCartesianOffsetUnits=m  TranslationStandardAxis=+Z  TranslationStandardOffset=0  TranslationStandardOffsetUnits=m  TranslationROffset=0  TranslationROffsetUnits=m  TranslationThetaOffset=0  TranslationThetaOffsetUnits=deg  TranslationZOffset=0  TranslationZOffsetUnits=m
  Memory : Memory
  PS-Simulink Converter1 : nesl_utility/PS-Simulink Converter  PhysicalDomain=network_engine_domain  SubClassName=ps_output  LeftPortType=input  RightPortType=output  PseudoPeriodic=off  Frequencies=[]  VectorFormat=inherit  Unit=inherit  AffineConversion=off
  PS-Simulink Converter3 : nesl_utility/PS-Simulink Converter  Commented=on  PhysicalDomain=network_engine_domain  SubClassName=ps_output  LeftPortType=input  RightPortType=output  PseudoPeriodic=off  Frequencies=[]  VectorFormat=inherit  Unit=inherit  AffineConversion=off
  PS-Simulink Converter4 : nesl_utility/PS-Simulink Converter  PhysicalDomain=network_engine_domain  SubClassName=ps_output  LeftPortType=input  RightPortType=output  PseudoPeriodic=off  Frequencies=[]  VectorFormat=inherit  Unit=inherit  AffineConversion=off
  PS-Simulink Converter5 : nesl_utility/PS-Simulink Converter  PhysicalDomain=network_engine_domain  SubClassName=ps_output  LeftPortType=input  RightPortType=output  PseudoPeriodic=off  Frequencies=[]  VectorFormat=inherit  Unit=inherit  AffineConversion=off
  PS-Simulink Converter6 : nesl_utility/PS-Simulink Converter  Commented=on  PhysicalDomain=network_engine_domain  SubClassName=ps_output  LeftPortType=input  RightPortType=output  PseudoPeriodic=off  Frequencies=[]  VectorFormat=inherit  Unit=inherit  AffineConversion=off
  Product : Product
  Product1 : Product
  Scope : Scope
  Simulink-PS Converter : nesl_utility/Simulink-PS Converter  PhysicalDomain=network_engine_domain  SubClassName=ps_input  LeftPortType=input  RightPortType=output  PseudoPeriodic=off  Frequencies=[]  NoiseDistribution=none  NoiseParameters=[]  Unit=1  AffineConversion=off  FilteringAndDerivatives=provide  SimscapeFilterOrder=1  InputFilterTimeConstant=0.001  UdotUserProvided=0
  Simulink-PS Converter1 : nesl_utility/Simulink-PS Converter  PhysicalDomain=network_engine_domain  SubClassName=ps_input  LeftPortType=input  RightPortType=output  PseudoPeriodic=off  Frequencies=[]  NoiseDistribution=none  NoiseParameters=[]  Unit=1  AffineConversion=off  FilteringAndDerivatives=provide  SimscapeFilterOrder=1  InputFilterTimeConstant=0.001  UdotUserProvided=0
  Simulink-PS Converter4 : nesl_utility/Simulink-PS Converter  Commented=on  PhysicalDomain=network_engine_domain  SubClassName=ps_input  LeftPortType=input  RightPortType=output  PseudoPeriodic=off  Frequencies=[]  NoiseDistribution=none  NoiseParameters=[]  Unit=1  AffineConversion=off  FilteringAndDerivatives=provide  SimscapeFilterOrder=1  InputFilterTimeConstant=0.001  UdotUserProvided=0
  Switch : Switch  Criteria=u2 > Threshold  SaturateOnIntegerOverflow=off  InputSameDT=off
  Transform Sensor : sm_lib/Frames and Transforms/Transform Sensor  MeasurementFrame=World  RotationSequence=XYX  SenseAngle=off  SenseAxis=off  SenseQ=off  SenseR=off  SenseRotationSequence=off  SenseOmegaX=off  SenseOmegaY=off  SenseOmegaZ=off  SenseOmega=off  SenseQDot=off  SenseRDot=off  SenseRotationSequenceDot=off  SenseAlphaX=off  SenseAlphaY=off  SenseAlphaZ=off  SenseAlpha=off  SenseQDDot=off  SenseRDDot=off  SenseX=off  SenseY=off  SenseZ=off  SenseXYZ=off  SenseRad=off  SenseAzim=off  SenseDist=off  SenseInc=off  SenseXDot=on  SenseYDot=on  SenseZDot=on  SenseXYZDot=off  SenseRadDot=off  SenseAzimDot=off  SenseDistDot=off  SenseIncDot=off  SenseXDDot=off  SenseYDDot=off  SenseZDDot=off  SenseXYZDDot=off  SenseRadDDot=off  SenseAzimDDot=off  SenseDistDDot=off  SenseIncDDot=off
  Transform Sensor1 : sm_lib/Frames and Transforms/Transform Sensor  MeasurementFrame=World  RotationSequence=XYX  SenseAngle=off  SenseAxis=off  SenseQ=off  SenseR=on  SenseRotationSequence=off  SenseOmegaX=off  SenseOmegaY=off  SenseOmegaZ=off  SenseOmega=off  SenseQDot=off  SenseRDot=off  SenseRotationSequenceDot=off  SenseAlphaX=off  SenseAlphaY=off  SenseAlphaZ=off  SenseAlpha=off  SenseQDDot=off  SenseRDDot=off  SenseX=off  SenseY=off  SenseZ=off  SenseXYZ=off  SenseRad=off  SenseAzim=off  SenseDist=off  SenseInc=off  SenseXDot=off  SenseYDot=on  SenseZDot=off  SenseXYZDot=off  SenseRadDot=off  SenseAzimDot=off  SenseDistDot=off  SenseIncDot=off  SenseXDDot=off  SenseYDDot=on  SenseZDDot=off  SenseXYZDDot=off  SenseRadDDot=off  SenseAzimDDot=off  SenseDistDDot=off  SenseIncDDot=off
  Transform Sensor2 : sm_lib/Frames and Transforms/Transform Sensor  MeasurementFrame=World  RotationSequence=XYX  SenseAngle=off  SenseAxis=off  SenseQ=off  SenseR=off  SenseRotationSequence=off  SenseOmegaX=off  SenseOmegaY=off  SenseOmegaZ=off  SenseOmega=off  SenseQDot=off  SenseRDot=off  SenseRotationSequenceDot=off  SenseAlphaX=off  SenseAlphaY=off  SenseAlphaZ=off  SenseAlpha=off  SenseQDDot=off  SenseRDDot=off  SenseX=off  SenseY=off  SenseZ=off  SenseXYZ=off  SenseRad=off  SenseAzim=off  SenseDist=off  SenseInc=off  SenseXDot=on  SenseYDot=on  SenseZDot=on  SenseXYZDot=off  SenseRadDot=off  SenseAzimDot=off  SenseDistDot=off  SenseIncDot=off  SenseXDDot=off  SenseYDDot=off  SenseZDDot=off  SenseXYZDDot=off  SenseRadDDot=off  SenseAzimDDot=off  SenseDistDDot=off  SenseIncDDot=off
  Transform Sensor3 : sm_lib/Frames and Transforms/Transform Sensor  MeasurementFrame=World  RotationSequence=XYX  SenseAngle=off  SenseAxis=off  SenseQ=off  SenseR=off  SenseRotationSequence=off  SenseOmegaX=off  SenseOmegaY=off  SenseOmegaZ=off  SenseOmega=off  SenseQDot=off  SenseRDot=off  SenseRotationSequenceDot=off  SenseAlphaX=off  SenseAlphaY=off  SenseAlphaZ=off  SenseAlpha=off  SenseQDDot=off  SenseRDDot=off  SenseX=off  SenseY=off  SenseZ=off  SenseXYZ=off  SenseRad=off  SenseAzim=off  SenseDist=off  SenseInc=off  SenseXDot=on  SenseYDot=on  SenseZDot=on  SenseXYZDot=off  SenseRadDot=off  SenseAzimDot=off  SenseDistDot=off  SenseIncDot=off  SenseXDDot=off  SenseYDDot=off  SenseZDDot=off  SenseXYZDDot=off  SenseRadDDot=off  SenseAzimDDot=off  SenseDistDDot=off  SenseIncDDot=off
  Varying Lowpass Filter : cstblocks/Linear Parameter Varying/Varying Lowpass Filter  N=2
  World Frame1 : sm_lib/Frames and Transforms/World Frame
  cutoff_freq(rad/s) : Constant  Value=noise_freq_cutoff
  h is positive when wing is low : Constant  Value=-1
  h is positive when wing is low1 : Constant  Value=-1
  pitch_lookup?(1=yes) : Constant  Value=pitch_lookup_input
  pitch_tip_in : FromWorkspace  VariableName=pitch_tip_in  SampleTime=del_t
  Cord2/4_F : PMIOPort  Side=Left
  dL : Outport
  dT : Outport  Port=2
  wires:
  [pitch_m] -> Switch/1
  pitch_tip_in/1 -> Switch/3  "pitch"
  pitch_lookup?(1=yes)/1 -> Switch/2
  cutoff_freq(rad/s)/1 -> Varying Lowpass Filter/2
  Memory/1 -> Varying Lowpass Filter/1
  Varying Lowpass Filter/1 -> AeroCalc/3(h_ddot)  "h_ddot_f"
  Product1/1 -> Memory/1  "h_ddot"
  PS-Simulink Converter1/1 -> Product1/1
  h is positive when wing is low1/1 -> Product1/2
  PS-Simulink Converter4/1 -> Product/1
  h is positive when wing is low/1 -> Product/2
  AeroCalc/3(stall_yes) -> Scope/1  "stall_if_positive"
  inboard_yes?/1 -> AeroCalc/5(in)
  Discrete Derivative1/1 -> AeroCalc/8(pitch_i_dd)
  Discrete Derivative/1 -> Discrete Derivative1/1, AeroCalc/7(pitch_i_d)
  i/1 -> AeroCalc/4(i)
  Switch/1 -> Discrete Derivative/1, AeroCalc/6(pitch_i)
  PS-Simulink Converter5/1 -> AeroCalc/1(R)  "R"
  Product/1 -> AeroCalc/2(h_dot)  "h_dot"
  AeroCalc/2(dT) -> Simulink-PS Converter1/1, dT/1  "dT"
  AeroCalc/1(dL) -> Simulink-PS Converter/1, dL/1  "dL"
  connections:
  Transform Sensor1/RConn4 -- PS-Simulink Converter1/LConn1
  Simulink-PS Converter1/RConn1 -- External Force and Torque1/LConn2
  F3/4/RConn1 -- Transform Sensor3/RConn1
  F1/4/RConn1 -- Transform Sensor/RConn1
  LeadingEdge/RConn1 -- Transform Sensor1/RConn1
  Transform Sensor1/RConn2 -- PS-Simulink Converter5/LConn1
  PS-Simulink Converter4/LConn1 -- Transform Sensor1/RConn3
  Transform Sensor2/RConn1 -- F3/4/LConn1 -- Cord2/4_F/RConn1 -- LeadingEdge/LConn1 -- F1/4/LConn1 -- External Force and Torque1/RConn1
  Simulink-PS Converter/RConn1 -- External Force and Torque1/LConn1
  Transform Sensor/LConn1 -- Transform Sensor2/LConn1 -- Transform Sensor3/LConn1 -- World Frame1/RConn1 -- Transform Sensor1/LConn1
